simulink model "con_nonlin"  (R2020b)
settings: Solver=VariableStepAuto  StartTime=0.0  StopTime=50.0  RelTol=1e-3
values from neighbouring files (symbols this model uses):
  alpha = 0.95    [main.m]
  amp = 0.3    [main.m]
  Ts = 0.15    [main.m]
  u_equ = 0.16    [main.m]
  x_equ = [0.2; 0]    [main.m]
settings Model: Creator=soren  LastModifiedBy=soren

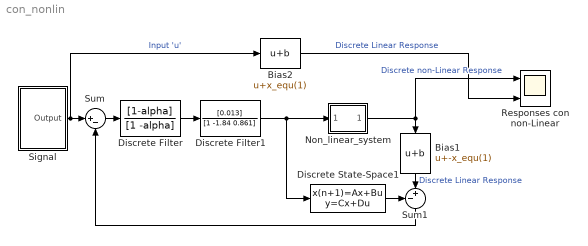
== system con_nonlin ==
  Bias1 : Bias  Bias=-x_equ(1)
  Bias2 : Bias  Bias=x_equ(1)
  Discrete Filter : DiscreteFilter  Numerator=[1-alpha]  Denominator=[1 -alpha]
  Discrete Filter1 : DiscreteFilter  Numerator=[0.013]  Denominator=[1 -1.84 0.861]
  Discrete State-Space1 : DiscreteStateSpace  A=[1 Ts;-3/4*Ts 1-Ts]  B=[0; 1.25*Ts]  C=[1, 0]  D=0  SampleTime=Ts
  Non_linear_system : Subsystem
  Responses con non-Linear : Scope  NumInputPorts=2
  Signal : Subsystem
  Sum : Sum  Inputs=|+-
  Sum1 : Sum  Inputs=-+|
  wires:
  Discrete Filter1/1 -> Non_linear_system/1(Input), Discrete State-Space1/1
  Bias2/1 -> Responses con non-Linear/2  "Discrete Linear Response"
  Bias1/1 -> Sum1/2  "Discrete Linear Response"
  Non_linear_system/1(Output) -> Responses con non-Linear/1, Bias1/1  "Discrete non-Linear Response"
  Discrete Filter/1 -> Discrete Filter1/1
  Discrete State-Space1/1 -> Sum1/1
  Signal/1(Output) -> Bias2/1, Sum/1  "Input 'u'"
  Sum/1 -> Discrete Filter/1
  Sum1/1 -> Sum/2

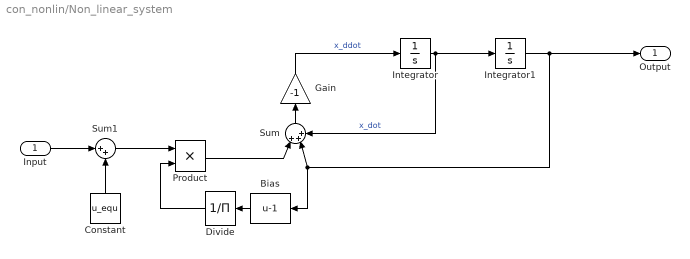
== system con_nonlin/Non_linear_system ==
  Input : Inport
  Bias : Bias  Bias=-1
  Constant : Constant  Value=u_equ
  Divide : Product  Inputs=/
  Gain : Gain  Gain=-1
  Integrator : Integrator
  Integrator1 : Integrator  InitialCondition=x_equ(1)
  Product : Product
  Sum : Sum  Inputs=|+++
  Sum1 : Sum  Inputs=|++
  Output : Outport
  wires:
  Integrator/1 -> Sum/3, Integrator1/1  "x_dot"
  Gain/1 -> Integrator/1  "x_ddot"
  Constant/1 -> Sum1/2
  Input/1 -> Sum1/1
  Integrator1/1 -> Output/1, Bias/1, Sum/2
  Bias/1 -> Divide/1
  Sum/1 -> Gain/1
  Sum1/1 -> Product/1
  Product/1 -> Sum/1
  Divide/1 -> Product/2

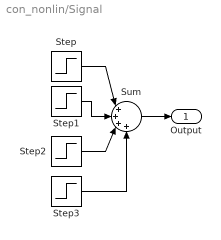
== system con_nonlin/Signal ==
  Step : Step  Time=10  After=0.2*amp  SampleTime=0
  Step1 : Step  Time=20  After=-0.2*amp  SampleTime=0
  Step2 : Step  Time=30  After=-0.2*amp  SampleTime=0
  Step3 : Step  Time=40  After=0.2*amp  SampleTime=0
  Sum : Sum  Inputs=|++++
  Output : Outport
  wires:
  Sum/1 -> Output/1
  Step2/1 -> Sum/3
  Step/1 -> Sum/1
  Step1/1 -> Sum/2
  Step3/1 -> Sum/4
